simulink model "simulinklab12"  (R2022b)
settings: Solver=VariableStepAuto  StartTime=0  StopTime=t_simulation  MaxStep=0.1  RelTol=1e-3
values from neighbouring files (symbols this model uses):
  Cvp = cp * rop * Vp    (= 90000)    [matlablab12.m]    (also in zajeciatermin7matalb.m)
  Cvw = cp * rop * Vw    (= 150000)    [matlablab12.m]    (also in zajeciatermin7matalb.m)
  dTzad = 3    [matlablab12.m]    (also in zajeciatermin7matalb.m = 5)
  Kcp = (qgN*a*(TwewN-TpN))/((TwewN * (1 + a) - TzewN - a*TpN)  * (TpN - TzewN))    (= 19.6078431373)    [matlablab12.m]    (also in zajeciatermin7matalb.m)
  Kcw = qgN/(TwewN * (1 + a) - TzewN - a * TpN)    (= 235.294117647)    [matlablab12.m]    (also in zajeciatermin7matalb.m)
  Kcwp = a*qgN/(TwewN*(1+a) -TzewN - a*TpN)    (= 58.8235294118)    [matlablab12.m]    (also in zajeciatermin7matalb.m)
  Tp0 = ((Kcw + Kcwp)*Kcp*Tzew0 + Kcwp*(qg0 + Kcw*Tzew0))/(Kcw*(Kcwp + Kcp) + Kcwp*Kcp)    (= 10)    [matlablab12.m]    (also in zajeciatermin7matalb.m)
  tskok = t_simulation/20    (= 1000)    [matlablab12.m]
  tskok2 = tskok *  6    (= 6000)    [matlablab12.m]
  Twew0 = (qg0*(Kcwp + Kcp) + Tzew0*(Kcw*Kcwp + Kcw * Kcp + Kcwp * Kcp))/(Kcw*(Kcwp + Kcp) + Kcwp * Kcp)    (= 20)    [matlablab12.m]    (also in zajeciatermin7matalb.m)
  Tzad = TpN    (= 10)    [matlablab12.m]    (also in zajeciatermin7matalb.m)
  Tzew0 = TzewN    (= -20)    [matlablab12.m]    (also in zajeciatermin7matalb.m)
libraries: slpidlib x3
settings Model: Creator=huber  LastModifiedBy=huber
settings DataIOCC: SaveFormat=StructureWithTime  ReturnWorkspaceOutputs=off
settings OptimizationCC: BlockReduction=off  BufferReuse=off
settings DebuggingCC: AlgebraicLoopMsg=none

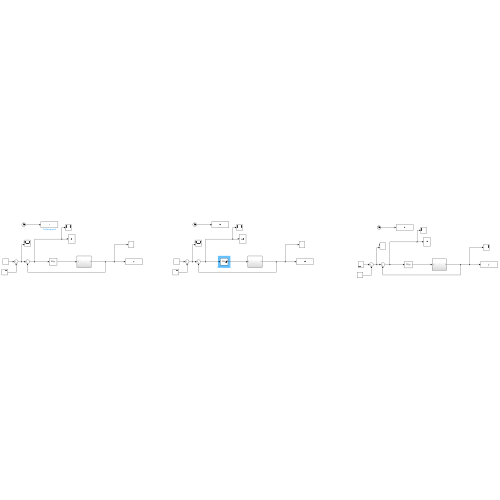
[thumbnail: Simulink's stored preview of the top-level diagram]
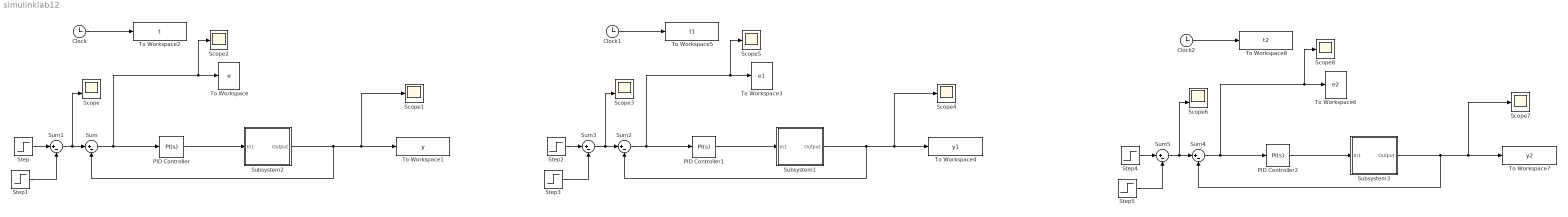
== system simulinklab12 ==
  Clock : Clock
  Clock1 : Clock
  Clock2 : Clock
  PID Controller : slpidlib/PID Controller  Controller=PI  Form=Parallel  TimeDomain=Continuous-time  UseExternalTs=off  SampleTime=-1  IntegratorMethod=Forward Euler  FilterMethod=Forward Euler  ControllerParametersSource=internal  P=6281.38247178475  I=0.548538951468863  UseKiTs=off  D=0  N=100  UseFilter=on  TunerSelectOption=Transfer Function Based (PID Tuner App)  InitialConditionSource=internal  InitialConditionForIntegrator=qg0  InitialConditionForFilter=0  DifferentiatorICPrevScaledInput=0  ExternalReset=none  TrackingMode=off  Kt=1  LimitOutput=off  SatLimitsSource=internal  UpperSaturationLimit=inf  LowerSaturationLimit=-inf  LinearizeAsGain=on  AntiWindupMode=none  Kb=1  LimitIntegrator=off  UpperIntegratorSaturationLimit=inf  LowerIntegratorSaturationLimit=-inf  POutMin=[]  POutMax=[]  IOutMin=[]  IOutMax=[]  DOutMin=[]  DOutMax=[]  NOutMin=[]  NOutMax=[]  SumOutMin=[]  SumOutMax=[]  SaturationOutMin=[]  SaturationOutMax=[]  PParamMin=[]  PParamMax=[]  IParamMin=[]  IParamMax=[]  DParamMin=[]  DParamMax=[]  NParamMin=[]  NParamMax=[]  KbParamMin=[]  KbParamMax=[]  KtParamMin=[]  KtParamMax=[]  KbOutMin=[]  KbOutMax=[]  KtOutMin=[]  KtOutMax=[]  IntegratorOutMin=[]  IntegratorOutMax=[]  FilterOutMin=[]  FilterOutMax=[]  SumI1OutMin=[]  SumI1OutMax=[]  SumI2OutMin=[]  SumI2OutMax=[]  SumI3OutMin=[]  SumI3OutMax=[]  SumI4OutMin=[]  SumI4OutMax=[]  SumDOutMin=[]  SumDOutMax=[]  DifferentiatorOutMin=[]  DifferentiatorOutMax=[]  FilterDiffOutCoefMin=[]  FilterDiffOutCoefMax=[]  ReciprocalOutMin=[]  ReciprocalOutMax=[]  SumDenOutMin=[]  SumDenOutMax=[]  SumNumOutMin=[]  SumNumOutMax=[]  DivideOutMin=[]  DivideOutMax=[]  UdiffTsProdOutMin=[]  UdiffTsProdOutMax=[]  NTsProdOutMin=[]  NTsProdOutMax=[]  UintegralTsProdOutMin=[]  UintegralTsProdOutMax=[]  UngainTsProdOutMin=[]  UngainTsProdOutMax=[]  ClampingZeroOutDataTypeStr=Inherit: Inherit via back propagation  ClampingZeroOutMin=[]  ClampingZeroOutMax=[]  FilterDenConstantOutDataTypeStr=Inherit: Inherit via back propagation  FilterDenConstantOutMin=[]  FilterDenConstantOutMax=[]  PCopyOutDataTypeStr=Inherit: Inherit via back propagation  PCopyOutMin=[]  PCopyOutMax=[]  NCopyOutDataTypeStr=Inherit: Inherit via back propagation  NCopyOutMin=[]  NCopyOutMax=[]  IntegratorContinuousStateAttributes=''  IntegratorStateMustResolveToSignalObject=off  IntegratorRTWStateStorageClass=Auto  FilterContinuousStateAttributes=''  FilterStateMustResolveToSignalObject=off  FilterRTWStateStorageClass=Auto  ParallelPVariant=InternalParameters  IdealPVariant=Disabled  IVariant=InternalParameters  DVariant=InternalParameters  IntegratorVariant=Continuous  SatVariant=Disabled  AWVariant=Passthrough  PCopyVariant=Disabled  TRVariant=Disabled  FdbkBlocksVariant=Forward  IdealPFdbkVariant=Disabled  SatFdbkVariant=Disabled  DerivativeFilterVariant=ContFilter  NVariant=InternalParameters  NCopyVariant=Disabled  FilterICVariant=InternalICsFilter  IntegratorICVariant=InternalICs  ExternalResetVariant=Disabled  TRSumVariant=Passthrough  SumFdbkVariant=Disabled  SumVariant=Sum_PID  TsampFilterVariant=InternalTs  TsampNgainVariant=Passthrough  TsampIntegralVariant=Passthrough  ExternalSaturationOutDataTypeStr=Inherit: Same as second input
  PID Controller1 : slpidlib/PID Controller  Controller=PI  Form=Parallel  TimeDomain=Continuous-time  UseExternalTs=off  SampleTime=-1  IntegratorMethod=Forward Euler  FilterMethod=Forward Euler  ControllerParametersSource=internal  P=6281.38247178475  I=0.548538951468863  UseKiTs=off  D=0  N=100  UseFilter=on  TunerSelectOption=Transfer Function Based (PID Tuner App)  InitialConditionSource=internal  InitialConditionForIntegrator=qg0  InitialConditionForFilter=0  DifferentiatorICPrevScaledInput=0  ExternalReset=none  TrackingMode=off  Kt=1  LimitOutput=on  SatLimitsSource=internal  UpperSaturationLimit=inf  LowerSaturationLimit=-inf  LinearizeAsGain=on  AntiWindupMode=back-calculation  Kb=2000  LimitIntegrator=off  UpperIntegratorSaturationLimit=inf  LowerIntegratorSaturationLimit=-inf  POutMin=[]  POutMax=[]  IOutMin=[]  IOutMax=[]  DOutMin=[]  DOutMax=[]  NOutMin=[]  NOutMax=[]  SumOutMin=[]  SumOutMax=[]  SaturationOutMin=[]  SaturationOutMax=[]  PParamMin=[]  PParamMax=[]  IParamMin=[]  IParamMax=[]  DParamMin=[]  DParamMax=[]  NParamMin=[]  NParamMax=[]  KbParamMin=[]  KbParamMax=[]  KtParamMin=[]  KtParamMax=[]  KbOutMin=[]  KbOutMax=[]  KtOutMin=[]  KtOutMax=[]  IntegratorOutMin=[]  IntegratorOutMax=[]  FilterOutMin=[]  FilterOutMax=[]  SumI1OutMin=[]  SumI1OutMax=[]  SumI2OutMin=[]  SumI2OutMax=[]  SumI3OutMin=[]  SumI3OutMax=[]  SumI4OutMin=[]  SumI4OutMax=[]  SumDOutMin=[]  SumDOutMax=[]  DifferentiatorOutMin=[]  DifferentiatorOutMax=[]  FilterDiffOutCoefMin=[]  FilterDiffOutCoefMax=[]  ReciprocalOutMin=[]  ReciprocalOutMax=[]  SumDenOutMin=[]  SumDenOutMax=[]  SumNumOutMin=[]  SumNumOutMax=[]  DivideOutMin=[]  DivideOutMax=[]  UdiffTsProdOutMin=[]  UdiffTsProdOutMax=[]  NTsProdOutMin=[]  NTsProdOutMax=[]  UintegralTsProdOutMin=[]  UintegralTsProdOutMax=[]  UngainTsProdOutMin=[]  UngainTsProdOutMax=[]  ClampingZeroOutDataTypeStr=Inherit: Inherit via back propagation  ClampingZeroOutMin=[]  ClampingZeroOutMax=[]  FilterDenConstantOutDataTypeStr=Inherit: Inherit via back propagation  FilterDenConstantOutMin=[]  FilterDenConstantOutMax=[]  PCopyOutDataTypeStr=Inherit: Inherit via back propagation  PCopyOutMin=[]  PCopyOutMax=[]  NCopyOutDataTypeStr=Inherit: Inherit via back propagation  NCopyOutMin=[]  NCopyOutMax=[]  IntegratorContinuousStateAttributes=''  IntegratorStateMustResolveToSignalObject=off  IntegratorRTWStateStorageClass=Auto  FilterContinuousStateAttributes=''  FilterStateMustResolveToSignalObject=off  FilterRTWStateStorageClass=Auto  ParallelPVariant=InternalParameters  IdealPVariant=Disabled  IVariant=InternalParameters  DVariant=InternalParameters  IntegratorVariant=Continuous  SatVariant=Disabled  AWVariant=Passthrough  PCopyVariant=Disabled  TRVariant=Disabled  FdbkBlocksVariant=Forward  IdealPFdbkVariant=Disabled  SatFdbkVariant=Disabled  DerivativeFilterVariant=ContFilter  NVariant=InternalParameters  NCopyVariant=Disabled  FilterICVariant=InternalICsFilter  IntegratorICVariant=InternalICs  ExternalResetVariant=Disabled  TRSumVariant=Passthrough  SumFdbkVariant=Disabled  SumVariant=Sum_PID  TsampFilterVariant=InternalTs  TsampNgainVariant=Passthrough  TsampIntegralVariant=Passthrough  ExternalSaturationOutDataTypeStr=Inherit: Same as second input
  PID Controller2 : slpidlib/PID Controller  Controller=PI  Form=Parallel  TimeDomain=Continuous-time  UseExternalTs=off  SampleTime=-1  IntegratorMethod=Forward Euler  FilterMethod=Forward Euler  ControllerParametersSource=internal  P=6281.38247178475  I=0.548538951468863  UseKiTs=off  D=0  N=100  UseFilter=on  TunerSelectOption=Transfer Function Based (PID Tuner App)  InitialConditionSource=internal  InitialConditionForIntegrator=qg0  InitialConditionForFilter=0  DifferentiatorICPrevScaledInput=0  ExternalReset=none  TrackingMode=off  Kt=1  LimitOutput=off  SatLimitsSource=external  UpperSaturationLimit=inf  LowerSaturationLimit=-inf  LinearizeAsGain=on  AntiWindupMode=none  Kb=1  LimitIntegrator=on  UpperIntegratorSaturationLimit=inf  LowerIntegratorSaturationLimit=-inf  POutMin=[]  POutMax=[]  IOutMin=[]  IOutMax=[]  DOutMin=[]  DOutMax=[]  NOutMin=[]  NOutMax=[]  SumOutMin=[]  SumOutMax=[]  SaturationOutMin=[]  SaturationOutMax=[]  PParamMin=[]  PParamMax=[]  IParamMin=[]  IParamMax=[]  DParamMin=[]  DParamMax=[]  NParamMin=[]  NParamMax=[]  KbParamMin=[]  KbParamMax=[]  KtParamMin=[]  KtParamMax=[]  KbOutMin=[]  KbOutMax=[]  KtOutMin=[]  KtOutMax=[]  IntegratorOutMin=[]  IntegratorOutMax=[]  FilterOutMin=[]  FilterOutMax=[]  SumI1OutMin=[]  SumI1OutMax=[]  SumI2OutMin=[]  SumI2OutMax=[]  SumI3OutMin=[]  SumI3OutMax=[]  SumI4OutMin=[]  SumI4OutMax=[]  SumDOutMin=[]  SumDOutMax=[]  DifferentiatorOutMin=[]  DifferentiatorOutMax=[]  FilterDiffOutCoefMin=[]  FilterDiffOutCoefMax=[]  ReciprocalOutMin=[]  ReciprocalOutMax=[]  SumDenOutMin=[]  SumDenOutMax=[]  SumNumOutMin=[]  SumNumOutMax=[]  DivideOutMin=[]  DivideOutMax=[]  UdiffTsProdOutMin=[]  UdiffTsProdOutMax=[]  NTsProdOutMin=[]  NTsProdOutMax=[]  UintegralTsProdOutMin=[]  UintegralTsProdOutMax=[]  UngainTsProdOutMin=[]  UngainTsProdOutMax=[]  ClampingZeroOutDataTypeStr=Inherit: Inherit via back propagation  ClampingZeroOutMin=[]  ClampingZeroOutMax=[]  FilterDenConstantOutDataTypeStr=Inherit: Inherit via back propagation  FilterDenConstantOutMin=[]  FilterDenConstantOutMax=[]  PCopyOutDataTypeStr=Inherit: Inherit via back propagation  PCopyOutMin=[]  PCopyOutMax=[]  NCopyOutDataTypeStr=Inherit: Inherit via back propagation  NCopyOutMin=[]  NCopyOutMax=[]  IntegratorContinuousStateAttributes=''  IntegratorStateMustResolveToSignalObject=off  IntegratorRTWStateStorageClass=Auto  FilterContinuousStateAttributes=''  FilterStateMustResolveToSignalObject=off  FilterRTWStateStorageClass=Auto  ParallelPVariant=InternalParameters  IdealPVariant=Disabled  IVariant=InternalParameters  DVariant=InternalParameters  IntegratorVariant=Continuous  SatVariant=Disabled  AWVariant=Passthrough  PCopyVariant=Disabled  TRVariant=Disabled  FdbkBlocksVariant=Forward  IdealPFdbkVariant=Disabled  SatFdbkVariant=Disabled  DerivativeFilterVariant=ContFilter  NVariant=InternalParameters  NCopyVariant=Disabled  FilterICVariant=InternalICsFilter  IntegratorICVariant=InternalICs  ExternalResetVariant=Disabled  TRSumVariant=Passthrough  SumFdbkVariant=Disabled  SumVariant=Sum_PID  TsampFilterVariant=InternalTs  TsampNgainVariant=Passthrough  TsampIntegralVariant=Passthrough  ExternalSaturationOutDataTypeStr=Inherit: Same as second input
  Scope : Scope  NumInputPorts=2
  Scope{1..2,4..5,7..8} (6 alike) : Scope
  Scope3 : Scope  NumInputPorts=2
  Scope6 : Scope  NumInputPorts=2
  Step : Step  Time=tskok  Before=Tzad  After=Tzad + dTzad  SampleTime=0
  Step1 : Step  Time=tskok2  After=dTzad  SampleTime=0
  Step2 : Step  Time=tskok  Before=Tzad  After=Tzad + dTzad  SampleTime=0
  Step3 : Step  Time=tskok2  After=dTzad  SampleTime=0
  Step4 : Step  Time=tskok  Before=Tzad  After=Tzad + dTzad  SampleTime=0
  Step5 : Step  Time=tskok2  After=dTzad  SampleTime=0
  Subsystem1 : Subsystem
  Subsystem2 : Subsystem
  Subsystem3 : Subsystem
  Sum{,1..5} (6 alike) : Sum  Inputs=|+-
  To Workspace : ToWorkspace  VariableName=e  SampleTime=-1
  To Workspace1 : ToWorkspace  VariableName=y  SampleTime=-1
  To Workspace2 : ToWorkspace  VariableName=t  SampleTime=-1
  To Workspace3 : ToWorkspace  VariableName=e1  SampleTime=-1
  To Workspace4 : ToWorkspace  VariableName=y1  SampleTime=-1
  To Workspace5 : ToWorkspace  VariableName=t1  SampleTime=-1
  To Workspace6 : ToWorkspace  VariableName=e2  SampleTime=-1
  To Workspace7 : ToWorkspace  VariableName=y2  SampleTime=-1
  To Workspace8 : ToWorkspace  VariableName=t2  SampleTime=-1
  wires:
  Clock/1 -> To Workspace2/1
  Step/1 -> Sum1/1
  Sum1/1 -> Scope/2, Sum/1
  Step1/1 -> Sum1/2
  Subsystem2/1(Output) -> Sum/2, Scope1/1, To Workspace1/1
  Sum/1 -> PID Controller/1, Scope2/1, To Workspace/1
  PID Controller/1 -> Subsystem2/1(In1)
  PID Controller1/1 -> Subsystem1/1(In1)
  Step3/1 -> Sum3/2
  Sum3/1 -> Scope3/2, Sum2/1
  Clock1/1 -> To Workspace5/1
  Subsystem1/1(Output) -> Sum2/2, Scope4/1, To Workspace4/1
  Step2/1 -> Sum3/1
  Sum2/1 -> Scope5/1, To Workspace3/1, PID Controller1/1
  PID Controller2/1 -> Subsystem3/1(In1)
  Step5/1 -> Sum5/2
  Sum5/1 -> Scope6/2, Sum4/1
  Clock2/1 -> To Workspace8/1
  Subsystem3/1(Output) -> Sum4/2, Scope7/1, To Workspace7/1
  Step4/1 -> Sum5/1
  Sum4/1 -> Scope8/1, To Workspace6/1, PID Controller2/1

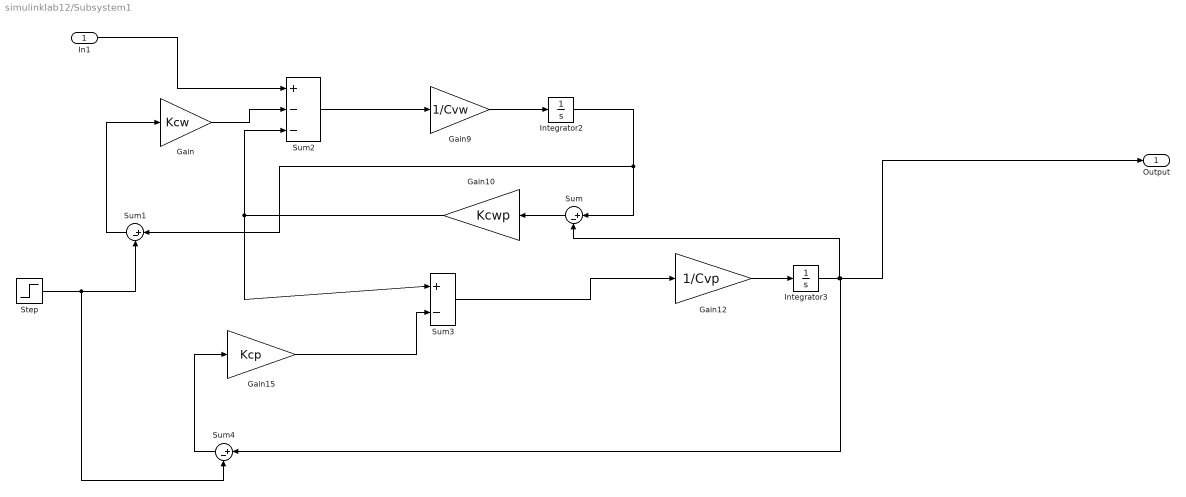
== system simulinklab12/Subsystem1 ==
  In1 : Inport
  Gain : Gain  Gain=Kcw
  Gain10 : Gain  Gain=Kcwp
  Gain12 : Gain  Gain=1/Cvp
  Gain15 : Gain  Gain=Kcp
  Gain9 : Gain  Gain=1/Cvw
  Integrator2 : Integrator  InitialCondition=Twew0
  Integrator3 : Integrator  InitialCondition=Tp0
  Step : Step  Time=tskok  Before=Tzew0  After=Tzew0 +Tzad  SampleTime=0
  Sum{,1,3..4} (4 alike) : Sum  Inputs=|+-
  Sum2 : Sum  Inputs=+--
  Output : Outport
  wires:
  Gain12/1 -> Integrator3/1
  Integrator2/1 -> Sum1/1, Sum/1
  Sum2/1 -> Gain9/1
  Gain9/1 -> Integrator2/1
  Gain10/1 -> Sum2/3, Sum3/1
  Integrator3/1 -> Output/1, Sum4/1, Sum/2
  Sum3/1 -> Gain12/1
  Gain15/1 -> Sum3/2
  In1/1 -> Sum2/1
  Step/1 -> Sum4/2, Sum1/2
  Gain/1 -> Sum2/2
  Sum1/1 -> Gain/1
  Sum/1 -> Gain10/1
  Sum4/1 -> Gain15/1

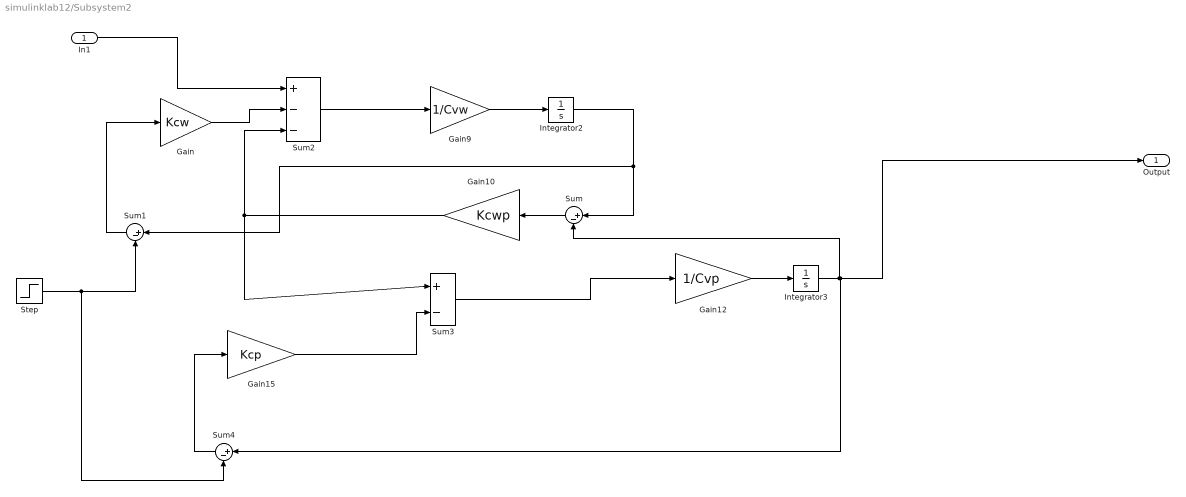
== system simulinklab12/Subsystem2 ==
  In1 : Inport
  Gain : Gain  Gain=Kcw
  Gain10 : Gain  Gain=Kcwp
  Gain12 : Gain  Gain=1/Cvp
  Gain15 : Gain  Gain=Kcp
  Gain9 : Gain  Gain=1/Cvw
  Integrator2 : Integrator  InitialCondition=Twew0
  Integrator3 : Integrator  InitialCondition=Tp0
  Step : Step  Time=tskok  Before=Tzew0  After=Tzew0 +Tzad  SampleTime=0
  Sum{,1,3..4} (4 alike) : Sum  Inputs=|+-
  Sum2 : Sum  Inputs=+--
  Output : Outport
  wires:
  Gain12/1 -> Integrator3/1
  Integrator2/1 -> Sum1/1, Sum/1
  Sum2/1 -> Gain9/1
  Gain9/1 -> Integrator2/1
  Gain10/1 -> Sum2/3, Sum3/1
  Integrator3/1 -> Output/1, Sum4/1, Sum/2
  Sum3/1 -> Gain12/1
  Gain15/1 -> Sum3/2
  In1/1 -> Sum2/1
  Step/1 -> Sum4/2, Sum1/2
  Gain/1 -> Sum2/2
  Sum1/1 -> Gain/1
  Sum/1 -> Gain10/1
  Sum4/1 -> Gain15/1

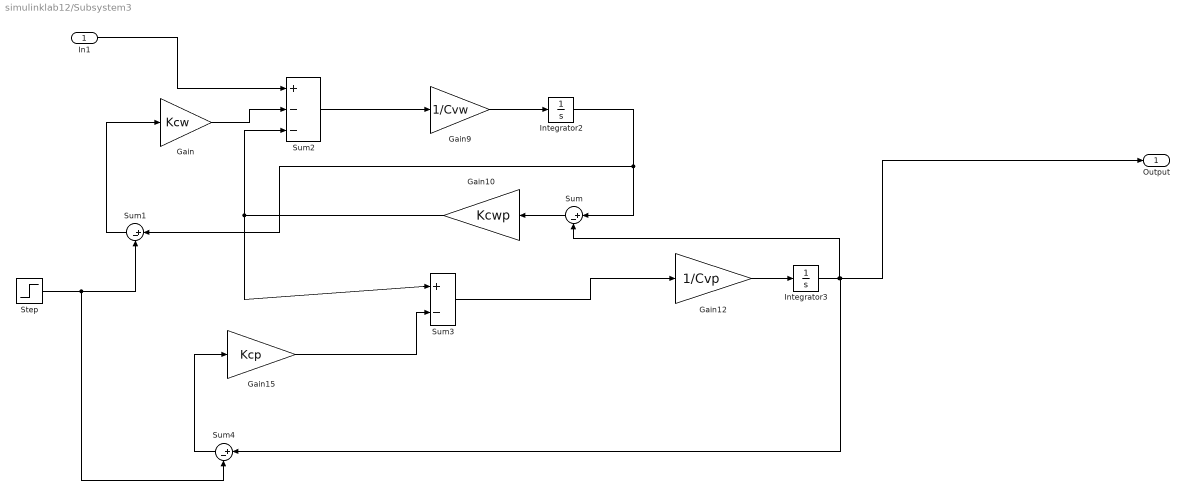
== system simulinklab12/Subsystem3 ==
  In1 : Inport
  Gain : Gain  Gain=Kcw
  Gain10 : Gain  Gain=Kcwp
  Gain12 : Gain  Gain=1/Cvp
  Gain15 : Gain  Gain=Kcp
  Gain9 : Gain  Gain=1/Cvw
  Integrator2 : Integrator  InitialCondition=Twew0
  Integrator3 : Integrator  InitialCondition=Tp0
  Step : Step  Time=tskok  Before=Tzew0  After=Tzew0 +Tzad  SampleTime=0
  Sum{,1,3..4} (4 alike) : Sum  Inputs=|+-
  Sum2 : Sum  Inputs=+--
  Output : Outport
  wires:
  Gain12/1 -> Integrator3/1
  Integrator2/1 -> Sum1/1, Sum/1
  Sum2/1 -> Gain9/1
  Gain9/1 -> Integrator2/1
  Gain10/1 -> Sum2/3, Sum3/1
  Integrator3/1 -> Output/1, Sum4/1, Sum/2
  Sum3/1 -> Gain12/1
  Gain15/1 -> Sum3/2
  In1/1 -> Sum2/1
  Step/1 -> Sum4/2, Sum1/2
  Gain/1 -> Sum2/2
  Sum1/1 -> Gain/1
  Sum/1 -> Gain10/1
  Sum4/1 -> Gain15/1
